simulink model "flipHDL_tb"  (R2024b)
settings: Solver=VariableStepAuto  StartTime=0.0  StopTime=10.0  RelTol=1e-3
settings Model: Creator=stefano  LastModifiedBy=stefano

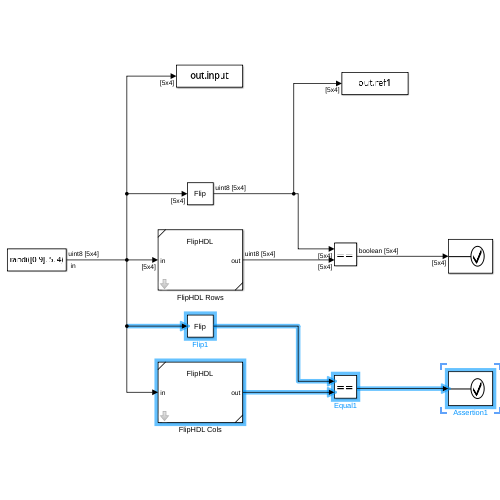
[thumbnail: Simulink's stored preview of the top-level diagram]
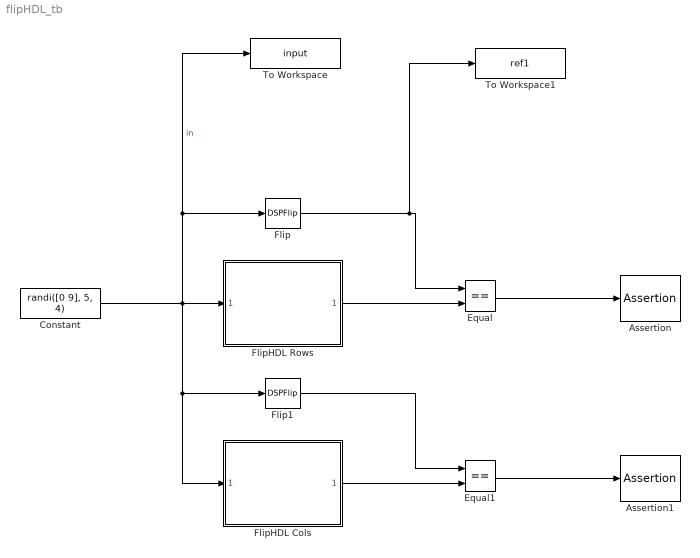
== system flipHDL_tb ==
  Assertion : Assertion  AssertionFailFcn="disp(\"Flip Along Rows assert fail\")"
  Assertion1 : Assertion  AssertionFailFcn="disp(\"Flip Along Columns assert fail\")"
  Constant : Constant  Value=randi([0 9], 5, 4)  VectorParams1D=off  OutDataTypeStr=uint8  SampleTime=1
  Equal : RelationalOperator  Operator===  OutDataTypeStr=boolean  RndMeth=Simplest  InputSameDT=off
  Equal1 : RelationalOperator  Operator===  OutDataTypeStr=boolean  RndMeth=Simplest  InputSameDT=off
  Flip : DSPFlip  dim=Rows
  Flip1 : DSPFlip
  FlipHDL Cols : Subsystem  ReferencedSubsystem=FlipHDL  flipAlong=Columns
  FlipHDL Rows : Subsystem  ReferencedSubsystem=FlipHDL  flipAlong=Rows
  To Workspace : ToWorkspace  VariableName=input  SaveFormat=Timeseries  SampleTime=-1
      settings: MaxDataPoints=1
  To Workspace1 : ToWorkspace  VariableName=ref1  SaveFormat=Timeseries  SampleTime=-1
      settings: MaxDataPoints=1
  wires:
  FlipHDL Rows/1 -> Equal/2
  Constant/1 -> To Workspace/1, Flip/1, FlipHDL Cols/1, Flip1/1, FlipHDL Rows/1  "in"
  Flip/1 -> To Workspace1/1, Equal/1
  Flip1/1 -> Equal1/1
  FlipHDL Cols/1 -> Equal1/2
  Equal/1 -> Assertion/1
  Equal1/1 -> Assertion1/1
